simulink model "setpoint_measurement"  (R2017a)
settings: Solver=FixedStepAuto  StartTime=0.0  StopTime=10.0  FixedStep=1/2048  RelTol=1e-3
settings Model: Creator=marce  LastModifiedBy=marce

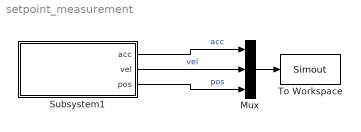
== system setpoint_measurement ==
  Mux : Mux  Inputs=3
  Subsystem1 : Subsystem  mask(Ref3){}
      settings: OpenFcn=r3g_main
      mask Display: disp('Ref3');
  To Workspace : ToWorkspace  VariableName=Simout  SaveFormat=Timeseries  SampleTime=-1
  wires:
  Mux/1 -> To Workspace/1
  Subsystem1/1(acc) -> Mux/1  "acc"
  Subsystem1/3(pos) -> Mux/3  "pos"
  Subsystem1/2(vel) -> Mux/2  "vel"

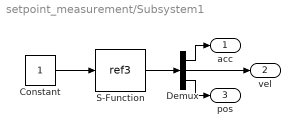
== system setpoint_measurement/Subsystem1 ==
  Constant : Constant
  Demux : Demux  Outputs=3
  S-Function : S-Function  FunctionName=ref3  Parameters=ref_part  SFunctionDeploymentMode=off  EnableBusSupport=off
      settings: OpenFcn=global ref_part; r3g_main
  acc : Outport
  vel : Outport  Port=2
  pos : Outport  Port=3
  wires:
  Constant/1 -> S-Function/1
  S-Function/1 -> Demux/1
  Demux/1 -> acc/1
  Demux/2 -> vel/1
  Demux/3 -> pos/1
